simulink model "DesignAwardEdition_CommentsImages"  (R2024b)
settings: Solver=FixedStepAuto  StartTime=0.0  StopTime=inf  RelTol=1e-3  EnableMultiTasking=on
libraries: vexarmcortexlib x22, vexcommonlib x3
settings Model: Creator=ierdn  LastModifiedBy=ierdn
settings DataIOCC: LimitDataPoints=on  SignalLoggingSaveFormat=ModelDataLogs  ReturnWorkspaceOutputs=off
settings OptimizationCC: ExpressionDepthLimit=2147483647  LifeSpan=Inf  MaxStackSize=64  EfficientTunableParamExpr=on
settings DebuggingCC: UnderspecifiedInitializationDetection=Classic  MergeDetectMultiDrivingBlocksExec=none  InheritedTsInSrcMsg=none  FcnCallInpInsideContextMsg=warning  StateNameClashWarn=warning  SFUnexpectedBacktrackingDiag=warning  SFNoUnconditionalDefaultTransitionDiag=warning  SFExecutionAtInitializationDiag=none  ArithmeticOperatorsInVariantConditions=warning
settings HardwareCC: ProdBitPerPointer=32  ProdBitPerSizeT=32  ProdBitPerPtrDiffT=32  ProdLargestAtomicInteger=Long  ProdLargestAtomicFloat=Double  ProdIntDivRoundTo=Undefined  ProdWordSize=32  ProdHWDeviceType=ARM Compatible->ARM Cortex
settings ModelReferenceCC: EnableRefExpFcnMdlSchedulingChecks=on  PropagateSignalLabelsOutOfModel=off
settings SFSimCC: MATLABDynamicMemAlloc=off  CustomCodeUndefinedFunction=UseInterfaceOnly
settings RTWCC: Description=Embedded Coder  SystemTargetFile=ert.tlc  HardwareBoard=ARM Cortex-based VEX Microcontroller  TemplateMakefile=ert_default_tmf  Toolchain=GNU Tools for VEX ARM Cortex  GPUComputeCapability=3.5
settings CodeAppCC: IgnoreCustomStorageClasses=off  CustomSymbolStrType=$N$R$M  StateflowObjectComments=on  InternalIdentifier=Classic
settings ERTTargetCC: CodeReplacementLibrary=GCC ARM Cortex-M3  MultiwordLength=2048  InlinedParameterPlacement=Hierarchical  ConvertIfToSwitch=off  SuppressUnreachableDefaultCases=off  DynamicArrayContainerType=coder::array

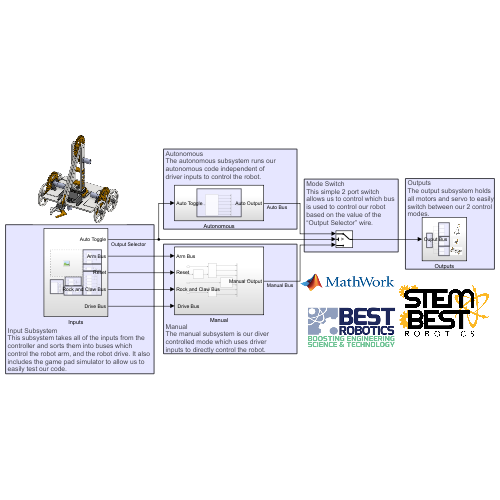
[thumbnail: Simulink's stored preview of the top-level diagram]
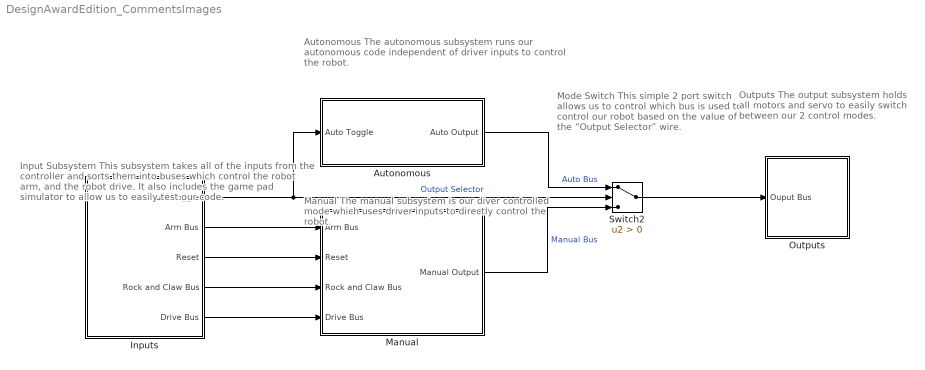
== system DesignAwardEdition_CommentsImages ==
  note: Input Subsystem
      | This subsystem takes all of the inputs from the
      | controller and sorts them into buses which
      | control the robot arm, and the robot drive. It also
      | includes the game pad simulator to allow us to
      | easily test our code.
  note: Mode Switch
      | This simple 2 port switch
      | allows us to control which bus
      | is used to control our robot
      | based on the value of the
      | “Output Selector” wire.
  note: Manual
      | The manual subsystem is our diver
      | controlled mode which uses driver
      | inputs to directly control the robot.
  note: Outputs
      | The output subsystem holds
      | all motors and servo to easily
      | switch between our 2 control
      | modes.
  note: Autonomous
      | The autonomous subsystem runs our
      | autonomous code independent of
      | driver inputs to control the robot.
  Autonomous : Subsystem
  Inputs : Subsystem
  Manual : Subsystem
  Outputs : Subsystem
  Switch2 : Switch  Criteria=u2 > Threshold  SaturateOnIntegerOverflow=off  InputSameDT=off
  wires:
  Inputs/1(Auto Toggle) -> Autonomous/1(Auto Toggle), Switch2/2  "Output Selector"
  Inputs/2(Arm Bus) -> Manual/1(Arm Bus)
  Inputs/3(Reset) -> Manual/2(Reset)
  Inputs/4(Rock and Claw Bus) -> Manual/3(Rock and Claw Bus)
  Inputs/5(" Drive Bus") -> Manual/4(" Drive Bus")
  Switch2/1 -> Outputs/1(Ouput Bus)
  Autonomous/1(Auto Output) -> Switch2/1  "Auto Bus"
  Manual/1(Manual Output) -> Switch2/3  "Manual Bus"

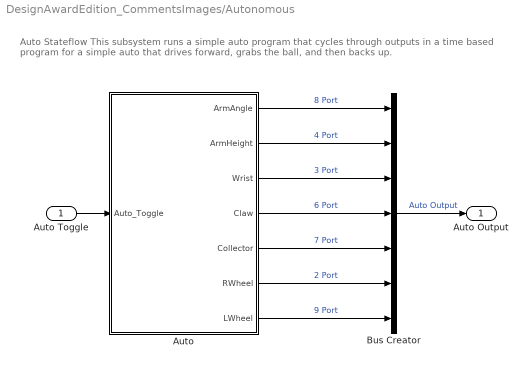
== system DesignAwardEdition_CommentsImages/Autonomous ==
  note: Auto Stateflow
      | This subsystem runs a simple auto program that cycles through outputs in a time based
      | program for a simple auto that drives forward, grabs the ball, and then backs up.
  Auto Toggle : Inport
  Auto : Stateflow chart  TreatAsAtomicUnit=on
      settings: PortSchema="{\"entries\":[{\"content\":{\"sides\":[{\"content\":{\"connectorIds\":[\"In1\"]},\"type\":\"ConnectorPlacement.EquallySpacedRectSide\",\"uuid\":\"cb75b4a7-821c-4b9c-9bc9-1f98599ada6a\"},{\"content\":{\"connectorIds\":[\"Out1\",\"Out2\",\"Out7\",\"Out3\",\"Out4\",\"Out5\",\"Out6\"],\"side\":\"RIGHT\"},\"type\":\"ConnectorPlacement.EquallySpacedRectSide\",\"uuid\":\"b2dd3252-08be-49f4-8f47-eb347fedf425\"},{\"content\":{\"side\":\"TOP\"},\"type\":\"ConnectorPlacement.EquallySpacedRectSide\",\"uuid\":\"9a4b743e-98c4-4195-adeb-f2b1f5e83854\"}]},\"type\":\"ConnectorPlacement.EquallySpacedConnector\",\"uuid\":\"cd3589b5-f3fd-437a-8269-f05dea4cca0b\"}],\"packageUris\":[\"http://schema.mathworks.com/mf0/Connector/R2020b\"],\"version\":\"1.0\"}"
  Bus Creator : BusCreator  Inputs=7
  Auto Output : Outport
  wires:
  Auto Toggle/1 -> Auto/1(Auto_Toggle)
  Bus Creator/1 -> Auto Output/1  "Auto Output"
  Auto/2(ArmHeight) -> Bus Creator/2  "4 Port"
  Auto/1(ArmAngle) -> Bus Creator/1  "8 Port"
  Auto/3(Claw) -> Bus Creator/4  "6 Port"
  Auto/4(Collector) -> Bus Creator/5  "7 Port"
  Auto/5(RWheel) -> Bus Creator/6  "2 Port"
  Auto/6(LWheel) -> Bus Creator/7  "9 Port"
  Auto/7(Wrist) -> Bus Creator/3  "3 Port"

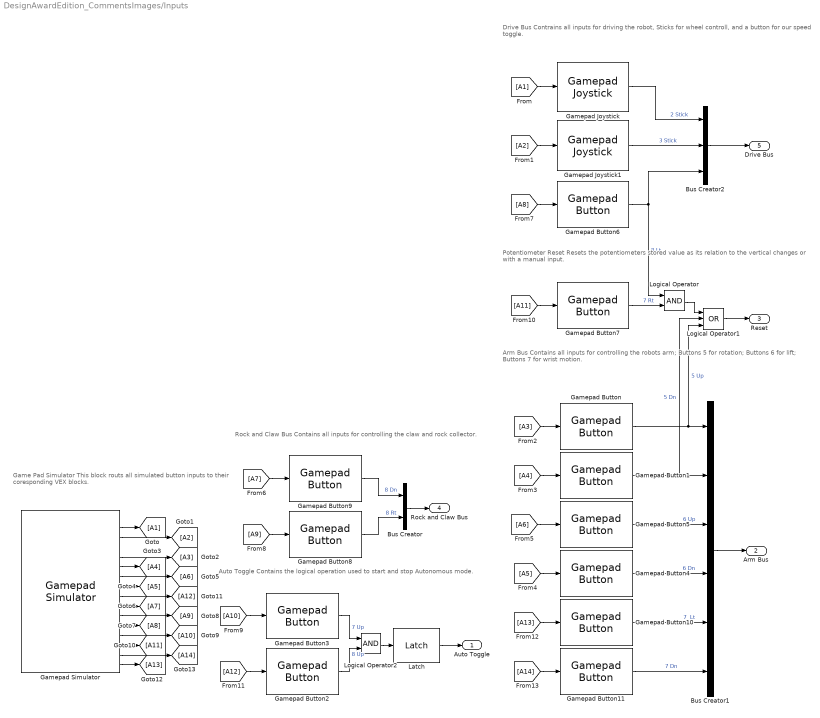
== system DesignAwardEdition_CommentsImages/Inputs ==
  note: Auto Toggle
      | Contains the logical operation used to start and stop Autonomous mode.
  note: Rock and Claw Bus
      | Contains all inputs for controlling the claw and rock collector.
  note: Game Pad Simulator
      | This block routs all simulated button inputs to their
      | coresponding VEX blocks.
  note: Arm Bus
      | Contains all inputs for controlling the robots arm;
      | Buttons 5 for rotation;
      | Buttons 6 for lift;
      | Buttons 7 for wrist motion.
  note: Potentiometer Reset
      | Resets the potentiometers stored value
      | as its relation to the vertical changes or
      | with a manual input.
  note: Drive Bus
      | Contrains all inputs for driving the robot, Sticks for wheel controll, and a button
      | for our speed toggle.
  Bus Creator : BusCreator  Inputs=2
  Bus Creator1 : BusCreator  Inputs=6
  Bus Creator2 : BusCreator  Inputs=3
  Gamepad Button : vexarmcortexlib/Gamepad/Gamepad Button  joystick=1  chan=5  button56=Up  button78=Down  SimulationIn=on  SampleTime=0.02
  Gamepad Button1 : vexarmcortexlib/Gamepad/Gamepad Button  joystick=1  chan=5  button56=Down  button78=Down  SimulationIn=on  SampleTime=0.02
  Gamepad Button10 : vexarmcortexlib/Gamepad/Gamepad Button  joystick=1  chan=7  button56=Up  button78=Left  SimulationIn=on  SampleTime=0.02
  Gamepad Button11 : vexarmcortexlib/Gamepad/Gamepad Button  joystick=1  chan=7  button56=Up  button78=Down  SimulationIn=on  SampleTime=0.02
  Gamepad Button2 : vexarmcortexlib/Gamepad/Gamepad Button  joystick=1  chan=8  button56=Up  button78=Up  SimulationIn=on  SampleTime=0.02
  Gamepad Button3 : vexarmcortexlib/Gamepad/Gamepad Button  joystick=1  chan=7  button56=Up  button78=Up  SimulationIn=on  SampleTime=0.02
  Gamepad Button4 : vexarmcortexlib/Gamepad/Gamepad Button  joystick=1  chan=6  button56=Down  button78=Down  SimulationIn=on  SampleTime=0.02
  Gamepad Button5 : vexarmcortexlib/Gamepad/Gamepad Button  joystick=1  chan=6  button56=Up  button78=Down  SimulationIn=on  SampleTime=0.02
  Gamepad Button6 : vexarmcortexlib/Gamepad/Gamepad Button  joystick=1  chan=8  button56=Up  button78=Left  SimulationIn=on  SampleTime=0.02
  Gamepad Button7 : vexarmcortexlib/Gamepad/Gamepad Button  joystick=1  chan=7  button56=Up  button78=Right  SimulationIn=on  SampleTime=0.02
  Gamepad Button8 : vexarmcortexlib/Gamepad/Gamepad Button  joystick=1  chan=8  button56=Up  button78=Right  SimulationIn=on  SampleTime=0.02
  Gamepad Button9 : vexarmcortexlib/Gamepad/Gamepad Button  joystick=1  chan=8  button56=Up  button78=Down  SimulationIn=on  SampleTime=0.02
  Gamepad Joystick : vexarmcortexlib/Gamepad/Gamepad Joystick  joystick=1  chan=2  SimulationIn=on  SampleTime=0.02
  Gamepad Joystick1 : vexarmcortexlib/Gamepad/Gamepad Joystick  joystick=1  chan=3  SimulationIn=on  SampleTime=0.02
  Gamepad Simulator : vexcommonlib/Gamepad Simulator  WhichPad=Logitech Gamepad  JoyId=1  BlockPlatform=vexarmcortex
      settings: LibrarySourceBlock=vexarmcortexlib/Utilities/Gamepad Simulator
  Latch : vexcommonlib/Latch  output0=off  BlockPlatform=vexarmcortex
      settings: LibrarySourceBlock=vexarmcortexlib/Utilities/Latch
  Logical Operator : Logic  AllPortsSameDT=off  OutDataTypeStr=boolean
  Logical Operator1 : Logic  Operator=OR  Inputs=3  AllPortsSameDT=off  OutDataTypeStr=boolean
  Logical Operator2 : Logic  AllPortsSameDT=off  OutDataTypeStr=boolean
  Auto Toggle : Outport
  Arm Bus : Outport  Port=2
  Reset : Outport  Port=3
  Rock and Claw Bus : Outport  Port=4
  " Drive Bus" : Outport  Port=5
  wires:
  Gamepad Button4/1 -> Bus Creator1/4  "6 Dn"
  Gamepad Button/1 -> Logical Operator1/3, Bus Creator1/1  "5 Up"
  Gamepad Button5/1 -> Bus Creator1/3  "6 Up"
  Gamepad Joystick/1 -> Bus Creator2/1  "2 Stick"
  Gamepad Joystick1/1 -> Bus Creator2/2  "3 Stick"
  Gamepad Button1/1 -> Logical Operator1/2, Bus Creator1/2  "5 Dn"
  Gamepad Button9/1 -> Bus Creator/1  "8 Dn"
  Gamepad Button8/1 -> Bus Creator/2  "8 Rt"
  Gamepad Button6/1 -> Logical Operator/1, Bus Creator2/3  "8 Lt"
  Gamepad Button7/1 -> Logical Operator/2  "7 Rt"
  Bus Creator2/1 -> " Drive Bus"/1
  Logical Operator/1 -> Logical Operator1/1
  Bus Creator1/1 -> Arm Bus/1
  Bus Creator/1 -> Rock and Claw Bus/1
  Logical Operator1/1 -> Reset/1
  Gamepad Simulator/2 -> [A1]
  [A1] -> Gamepad Joystick/1
  Gamepad Simulator/3 -> [A2]
  [A2] -> Gamepad Joystick1/1
  Gamepad Simulator/5 -> [A3]
  [A3] -> Gamepad Button/1
  Gamepad Simulator/6 -> [A4]
  [A4] -> Gamepad Button1/1
  Gamepad Simulator/8 -> [A5]
  [A5] -> Gamepad Button4/1
  Gamepad Simulator/7 -> [A6]
  [A6] -> Gamepad Button5/1
  Gamepad Simulator/10 -> [A7]
  [A7] -> Gamepad Button9/1
  Gamepad Simulator/12 -> [A8]
  [A8] -> Gamepad Button6/1
  Gamepad Simulator/11 -> [A9]
  [A9] -> Gamepad Button8/1
  [A10] -> Gamepad Button3/1
  Gamepad Simulator/14 -> [A11]
  [A11] -> Gamepad Button7/1
  Gamepad Simulator/9 -> [A12]
  [A12] -> Gamepad Button2/1
  Gamepad Button3/1 -> Logical Operator2/1  "7 Up"
  Gamepad Button2/1 -> Logical Operator2/2  "8 Up"
  Logical Operator2/1 -> Latch/1
  Latch/1 -> Auto Toggle/1
  Gamepad Simulator/13 -> [A10]
  Gamepad Simulator/16 -> [A13]
  [A13] -> Gamepad Button10/1
  Gamepad Simulator/15 -> [A14]
  [A14] -> Gamepad Button11/1
  Gamepad Button10/1 -> Bus Creator1/5  "7  Lt"
  Gamepad Button11/1 -> Bus Creator1/6  "7 Dn"

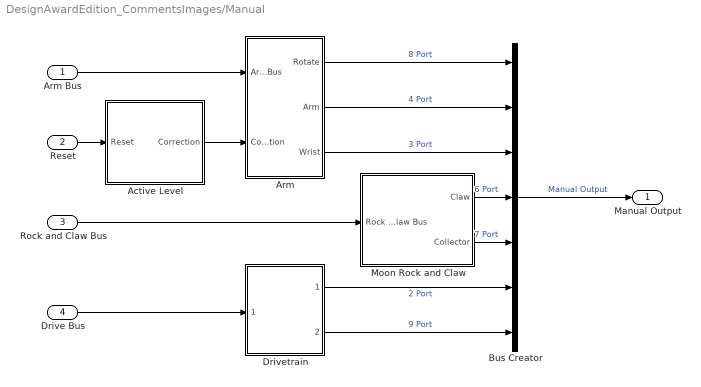
== system DesignAwardEdition_CommentsImages/Manual ==
  Arm Bus : Inport
  Reset : Inport  Port=2
  Rock and Claw Bus : Inport  Port=3
  " Drive Bus" : Inport  Port=4
  Active Level : Subsystem
  Arm : Subsystem
  Bus Creator : BusCreator  Inputs=7
  Drivetrain : Subsystem
  Moon Rock and Claw : Subsystem
  Manual Output : Outport
  wires:
  Active Level/1(Correction) -> Arm/2(Correction)
  Arm/2(Arm) -> Bus Creator/2  "4 Port"
  Moon Rock and Claw/2(Collector) -> Bus Creator/5  "7 Port"
  Drivetrain/1(Right Wheel) -> Bus Creator/6  "2 Port"
  Drivetrain/2(Left Wheel) -> Bus Creator/7  "9 Port"
  Arm/1(Rotate) -> Bus Creator/1  "8 Port"
  Arm/3(Wrist) -> Bus Creator/3  "3 Port"
  Moon Rock and Claw/1(Claw) -> Bus Creator/4  "6 Port"
  Rock and Claw Bus/1 -> Moon Rock and Claw/1(Rock and Claw Bus)
  Reset/1 -> Active Level/1(Reset)
  " Drive Bus"/1 -> Drivetrain/1(" Drive Bus")
  Arm Bus/1 -> Arm/1(Arm Bus)
  Bus Creator/1 -> Manual Output/1  "Manual Output"

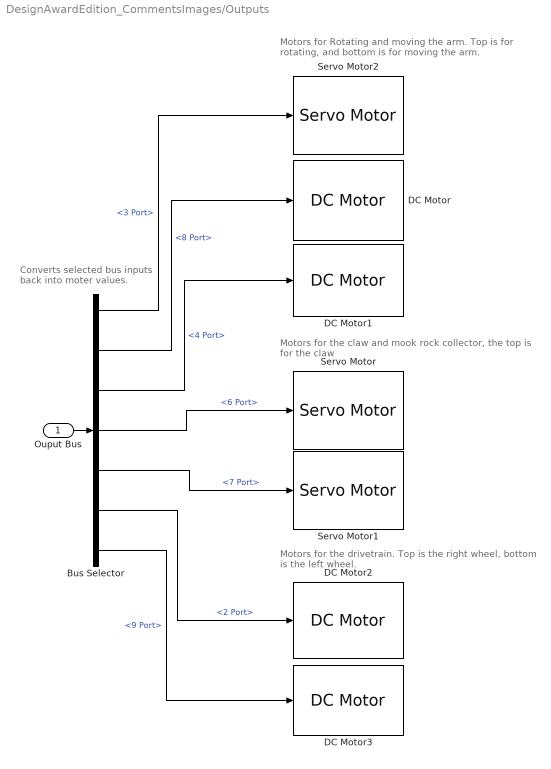
== system DesignAwardEdition_CommentsImages/Outputs ==
  note: Converts selected bus
      | inputs back into moter
      | values.
  note: Motors for Rotating and moving the arm.
      | Top is for rotating, and bottom is for moving the arm.
  note: Motors for the claw and mook rock
      | collector, the top is for the claw
  note: Motors for the drivetrain. Top is the right
      | wheel, bottom is the left wheel.
  Ouput Bus : Inport
  Bus Selector : BusSelector  OutputSignals=3 Port,8 Port,4 Port,6 Port,7 Port,2 Port,9 Port
  DC Motor : vexarmcortexlib/Actuators/DC Motor  motor=8  scaleFactor=1/13.5  SimulationOut=off
  DC Motor1 : vexarmcortexlib/Actuators/DC Motor  motor=4  scaleFactor=1/13.5  SimulationOut=off
  DC Motor2 : vexarmcortexlib/Actuators/DC Motor  motor=2  scaleFactor=1/13.5  SimulationOut=off
  DC Motor3 : vexarmcortexlib/Actuators/DC Motor  motor=9  scaleFactor=1/13.5  SimulationOut=off
  Servo Motor : vexarmcortexlib/Actuators/Servo Motor  motor=6  scaleFactor=60/127  SimulationOut=off
  Servo Motor1 : vexarmcortexlib/Actuators/Servo Motor  motor=7  scaleFactor=60/127  SimulationOut=off
  Servo Motor2 : vexarmcortexlib/Actuators/Servo Motor  motor=3  scaleFactor=60/127  SimulationOut=off
  wires:
  Ouput Bus/1 -> Bus Selector/1
  Bus Selector/2 -> DC Motor/1  "<8 Port>"
  Bus Selector/3 -> DC Motor1/1  "<4 Port>"
  Bus Selector/6 -> DC Motor2/1  "<2 Port>"
  Bus Selector/7 -> DC Motor3/1  "<9 Port>"
  Bus Selector/4 -> Servo Motor/1  "<6 Port>"
  Bus Selector/5 -> Servo Motor1/1  "<7 Port>"
  Bus Selector/1 -> Servo Motor2/1  "<3 Port>"

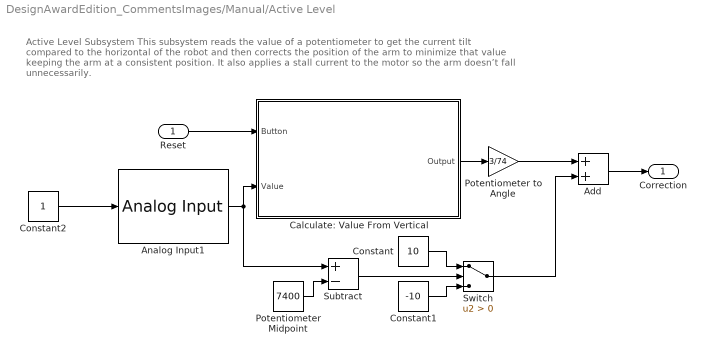
== system DesignAwardEdition_CommentsImages/Manual/Active Level ==
  note: Active Level Subsystem
      | This subsystem reads the value of a potentiometer to get the current tilt compared to the horizontal of the robot and then
      | corrects the position of the arm to minimize that value keeping the arm at a consistent position. It also applies a stall current
      | to the motor so the arm doesn’t fall unnecessarily.
  Reset : Inport
  Add : Sum
  Analog Input1 : vexarmcortexlib/Sensors/Analog Input  inChan=1  SimulationIn=on  SampleTime=0.02
  Calculate: Value From Vertical : Stateflow chart  TreatAsAtomicUnit=on
  Constant : Constant  Value=10
  Constant1 : Constant  Value=-10
  Constant2 : Constant
  Potentiometer Midpoint : Constant  Value=7400
  Potentiometer to Angle : Gain  Gain=3/74
  Subtract : Sum  Inputs=+-
  Switch : Switch  Criteria=u2 > Threshold  SaturateOnIntegerOverflow=off  InputSameDT=off
  Correction : Outport
  wires:
  Calculate: Value From Vertical/1(Output) -> Potentiometer to Angle/1
  Analog Input1/1 -> Subtract/1, Calculate: Value From Vertical/2(Value)
  Reset/1 -> Calculate: Value From Vertical/1(Button)
  Constant/1 -> Switch/1
  Constant1/1 -> Switch/3
  Potentiometer to Angle/1 -> Add/1
  Switch/1 -> Add/2
  Add/1 -> Correction/1
  Constant2/1 -> Analog Input1/1
  Subtract/1 -> Switch/2
  Potentiometer Midpoint/1 -> Subtract/2

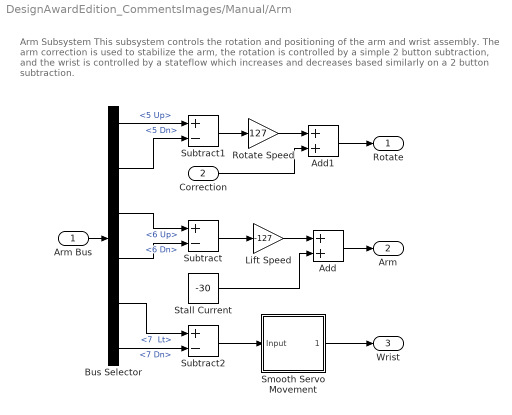
== system DesignAwardEdition_CommentsImages/Manual/Arm ==
  note: Arm Subsystem
      | This subsystem controls the rotation and positioning of the arm and wrist
      | assembly. The arm correction is used to stabilize the arm, the rotation is controlled
      | by a simple 2 button subtraction, and the wrist is controlled by a stateflow which
      | increases and decreases based similarly on a 2 button subtraction.
  Arm Bus : Inport
  Correction : Inport  Port=2
  Add : Sum
  Add1 : Sum
  Bus Selector : BusSelector  OutputSignals="5 Up,5 Dn,6 Up,6 Dn,7  Lt,7 Dn"
  Lift Speed : Gain  Gain=-127
  Rotate Speed : Gain  Gain=127
  Smooth Servo Movement : Stateflow chart  TreatAsAtomicUnit=on
  Stall Current : Constant  Value=-30
  Subtract : Sum  Inputs=+-
  Subtract1 : Sum  Inputs=+-
  Subtract2 : Sum  Inputs=+-
  Rotate : Outport
  Arm : Outport  Port=2
  Wrist : Outport  Port=3
  wires:
  Rotate Speed/1 -> Add1/1
  Add1/1 -> Rotate/1
  Stall Current/1 -> Add/2
  Subtract1/1 -> Rotate Speed/1
  Add/1 -> Arm/1
  Subtract/1 -> Lift Speed/1
  Lift Speed/1 -> Add/1
  Arm Bus/1 -> Bus Selector/1
  Correction/1 -> Add1/2
  Subtract2/1 -> Smooth Servo Movement/1(Input)
  Smooth Servo Movement/1(Output) -> Wrist/1
  Bus Selector/1 -> Subtract1/1  "<5 Up>"
  Bus Selector/2 -> Subtract1/2  "<5 Dn>"
  Bus Selector/3 -> Subtract/1  "<6 Up>"
  Bus Selector/4 -> Subtract/2  "<6 Dn>"
  Bus Selector/5 -> Subtract2/1  "<7  Lt>"
  Bus Selector/6 -> Subtract2/2  "<7 Dn>"

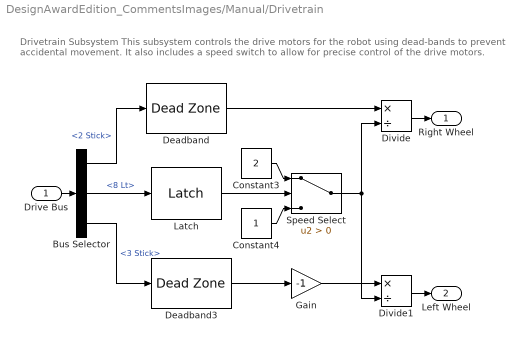
== system DesignAwardEdition_CommentsImages/Manual/Drivetrain ==
  note: Drivetrain Subsystem
      | This subsystem controls the drive motors for the robot using dead-bands to prevent
      | accidental movement. It also includes a speed switch to allow for precise control of
      | the drive motors.
  " Drive Bus" : Inport
  Bus Selector : BusSelector  OutputSignals=2 Stick,8 Lt,3 Stick
  Constant3 : Constant  Value=2
  Constant4 : Constant
  Deadband : DeadZone  LowerValue=-9  UpperValue=9
  Deadband3 : DeadZone  LowerValue=-9  UpperValue=9
  Divide : Product  Inputs=*/
  Divide1 : Product  Inputs=*/
  Gain : Gain  Gain=-1
  Latch : vexcommonlib/Latch  output0=off  BlockPlatform=vexarmcortex
  Speed Select : Switch  Criteria=u2 > Threshold  SaturateOnIntegerOverflow=off  InputSameDT=off
  Right Wheel : Outport
  Left Wheel : Outport  Port=2
  wires:
  Speed Select/1 -> Divide1/2, Divide/2
  Latch/1 -> Speed Select/2
  Constant3/1 -> Speed Select/1
  Deadband3/1 -> Gain/1
  Constant4/1 -> Speed Select/3
  Divide/1 -> Right Wheel/1
  Divide1/1 -> Left Wheel/1
  " Drive Bus"/1 -> Bus Selector/1
  Bus Selector/1 -> Deadband/1  "<2 Stick>"
  Bus Selector/3 -> Deadband3/1  "<3 Stick>"
  Bus Selector/2 -> Latch/1  "<8 Lt>"
  Deadband/1 -> Divide/1
  Gain/1 -> Divide1/1

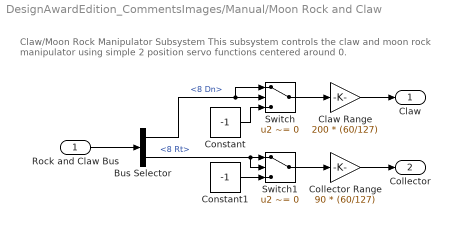
== system DesignAwardEdition_CommentsImages/Manual/Moon Rock and Claw ==
  note: Claw/Moon Rock Manipulator Subsystem
      | This subsystem controls the claw and moon rock manipulator using simple 2
      | position servo functions centered around 0.
  Rock and Claw Bus : Inport
  Bus Selector : BusSelector  OutputSignals=8 Dn,8 Rt
  Claw Range : Gain  Gain=200 * (60/127)
  Collector Range : Gain  Gain=90 * (60/127)
  Constant : Constant  Value=-1
  Constant1 : Constant  Value=-1
  Switch : Switch  Criteria=u2 ~= 0  SaturateOnIntegerOverflow=off  InputSameDT=off
  Switch1 : Switch  Criteria=u2 ~= 0  SaturateOnIntegerOverflow=off  InputSameDT=off
  Claw : Outport
  Collector : Outport  Port=2
  wires:
  Switch1/1 -> Collector Range/1
  Bus Selector/2 -> Switch1/2, Switch1/1  "<8 Rt>"
  Collector Range/1 -> Collector/1
  Constant1/1 -> Switch1/3
  Claw Range/1 -> Claw/1
  Switch/1 -> Claw Range/1
  Constant/1 -> Switch/3
  Rock and Claw Bus/1 -> Bus Selector/1
  Bus Selector/1 -> Switch/1, Switch/2  "<8 Dn>"

== stateflow chart DesignAwardEdition_CommentsImages/Manual/Active Level/Calculate: Value From Vertical ==
  state Calculate
    Output = Value - Stored;
  state Start
    Stored = Value;
    Output = 0;
  (default) -> Start
  Start -> Calculate : [Button == 0]
  Calculate -> Start : [Button == 1]
  data: Output output; Stored local; Button input; Value input

== stateflow chart DesignAwardEdition_CommentsImages/Manual/Arm/Smooth Servo Movement ==
  state Constant
    Speed = 3.5;
  state Change
    Output=Output+(Input*Speed);
  (default) -> Constant : {Output = 0}
  Constant -> Change : [(Input ~= 0)&&(Output >= -127 || Input == 1)&&(Output <= 127 || Input == -1)]
  Change -> Constant
  data: Input input; Output output; Speed local

== stateflow chart DesignAwardEdition_CommentsImages/Autonomous/Auto ==
  state Off
    LWheel = 0;
    RWheel = 0;
    Claw = -90;
    Collector = 0;
    ArmHeight = 0;
    ArmAngle = 0;
    Wrist = 0;
  state Approach
    LWheel = 50
    RWheel = 50
  state Grab
    LWheel = 0;
    RWheel = 0;
    Claw = 90;
  state Reverse
    LWheel = -50;
    RWheel = -50;
  (default) -> Off
  Reverse -> Off : [after(0.5,sec)]
  Off -> Approach : [Auto_Toggle == 1]
  Approach -> Grab : [after(0.5,sec)]
  Grab -> Reverse : [after(0.5,sec)]
  data: Auto_Toggle input; ArmAngle output; ArmHeight output; Claw output; Collector output; RWheel output; LWheel output; Wrist output
